simulink model "transform_ENU_to_NED"  (R2021a)
settings: Solver=FixedStepAuto  StartTime=0.0  StopTime=10.0  RelTol=1e-3
settings Model: Creator=esl  LastModifiedBy=esl
settings OptimizationCC: DefaultParameterBehavior=Inlined  GainParamInheritBuiltInType=on  UseFloatMulNetSlope=on  InlineInvariantSignals=on  ZeroExternalMemoryAtStartup=off  ZeroInternalMemoryAtStartup=off  EfficientFloat2IntCast=on  LifeSpan=1
settings HardwareCC: ProdLongLongMode=on
settings SFSimCC: MATLABDynamicMemAlloc=off
settings RTWCC: GenerateReport=on  LaunchReport=on  TargetLang=C++
settings CodeAppCC: ForceParamTrailComments=on
settings GRTTargetCC: TargetLangStandard=C++03 (ISO)  CombineSignalStateStructs=on  MatFileLogging=off  CodeInterfacePackaging=C++ class  SupportVariableSizeSignals=on

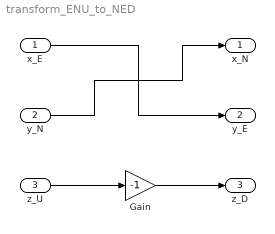
== system transform_ENU_to_NED ==
  x_E : Inport
  y_N : Inport  Port=2
  z_U : Inport  Port=3
  Gain : Gain  Gain=-1
  x_N : Outport
  y_E : Outport  Port=2
  z_D : Outport  Port=3
  wires:
  Gain/1 -> z_D/1
  z_U/1 -> Gain/1
  x_E/1 -> y_E/1
  y_N/1 -> x_N/1
